simulink model "uGrid_1PH_hd_caso2"  (R2017a)
settings: Solver=VariableStepAuto  StartTime=0.0  StopTime=5  FixedStep=1e-6  MaxStep=1e-4  RelTol=1e-3
PreLoadFcn:
  | SimulinkInit
InitFcn:
  | SimulinkInit
StartFcn:
  | SimulinkInit
StopFcn:
  | EndingScript
values from neighbouring files (symbols this model uses):
  J = 0.3    [SimulinkInit.m]
  K1 = 1.15    [SimulinkInit.m]
  K2 = 1    [SimulinkInit.m]
  K3 = 1    [SimulinkInit.m]
  P = 0.1    [SimulinkInit.m]
  Tao1 = 0.5    [SimulinkInit.m]
  Tao2 = 0.125    [SimulinkInit.m]
undefined symbols (not defined in the file or in its folder): G, GF, Ion, Lithium
libraries: powerlib x56, truetime x15, dsparch4 x12, powerlib_meascontrol x4, electricdrivelib x1, simulink x1
(part 2 of 2)

== system uGrid_1PH_hd_caso2/1Ph_Inverter_bio/Steper3 ==
  In1 : Inport
  Product : Product
  Step : Step  Time=st_time  SampleTime=samp_f
  Out1 : Outport
  wires:
  Product/1 -> Out1/1
  In1/1 -> Product/1
  Step/1 -> Product/2

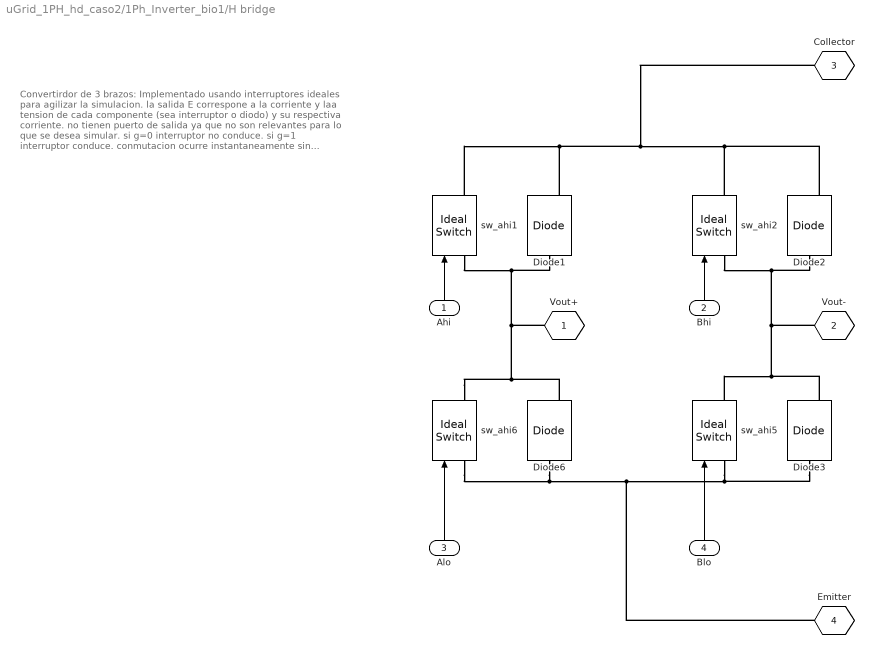
== system uGrid_1PH_hd_caso2/1Ph_Inverter_bio1/H bridge ==
  note: Convertirdor de 3 brazos:
      |
      | Implementado usando interruptores
      | ideales para agilizar la simulacion.
      | la salida E correspone a la corriente y laa
      | tension de cada componente
      | (sea interruptor o diodo) y su respectiva
      | corriente. no tienen puerto de salida ya que no
      | son relevantes para lo que se desea simular.
      |
      | si g=0 interruptor no conduce.
      | si g=1 interruptor conduce.
      |
      | conmutacion ocurre instantaneamente sin
      | retardo.
  Ahi : Inport
  Bhi : Inport  Port=2
  Alo : Inport  Port=3
  Blo : Inport  Port=4
   sw_ahi{1..2,5..6} (4 alike) : powerlib/Power Electronics/Ideal Switch  Ron=0.1  Lon=0  IC=0  Rs=1e6  Cs=10e-12  Measurements=on
  Diode{1..3,6} (4 alike) : powerlib/Power Electronics/Diode  Ron=.2  Lon=0  Vf=0.8  IC=0  UseSnubber=0  Rs=0  Cs=0  Measurements=on
  " Vout+" : PMIOPort  Tag=PMCPort  Port=1  Side=Right
  Vout- : PMIOPort  Tag=PMCPort  Port=2  Side=Right
  Collector : PMIOPort  Tag=PMCPort  Port=3  Side=Right
  Emitter : PMIOPort  Tag=PMCPort  Port=4  Side=Right
  wires:
  Alo/1 -> " sw_ahi6"/1
  Ahi/1 -> " sw_ahi1"/1
  Blo/1 -> " sw_ahi5"/1
  Bhi/1 -> " sw_ahi2"/1
  connections:
  Diode3/RConn1 -- Vout-/RConn1 -- " sw_ahi2"/LConn1 -- Diode2/LConn1 -- " sw_ahi5"/RConn1
  Diode3/LConn1 -- Emitter/RConn1 -- Diode6/LConn1 -- " sw_ahi6"/LConn1 -- " sw_ahi5"/LConn1
  Diode2/RConn1 -- Collector/RConn1 -- " sw_ahi1"/RConn1 -- Diode1/RConn1 -- " sw_ahi2"/RConn1
  " sw_ahi6"/RConn1 -- Diode6/RConn1 -- " Vout+"/RConn1 -- Diode1/LConn1 -- " sw_ahi1"/LConn1

== system uGrid_1PH_hd_caso2/1Ph_Inverter_bio1/Steper1 ==
  In1 : Inport
  Product : Product
  Step : Step  Time=st_time  SampleTime=samp_f
  Out1 : Outport
  wires:
  Step/1 -> Product/2
  In1/1 -> Product/1
  Product/1 -> Out1/1

== system uGrid_1PH_hd_caso2/1Ph_Inverter_bio1/Steper3 ==
  In1 : Inport
  Product : Product
  Step : Step  Time=st_time  SampleTime=samp_f
  Out1 : Outport
  wires:
  Product/1 -> Out1/1
  In1/1 -> Product/1
  Step/1 -> Product/2

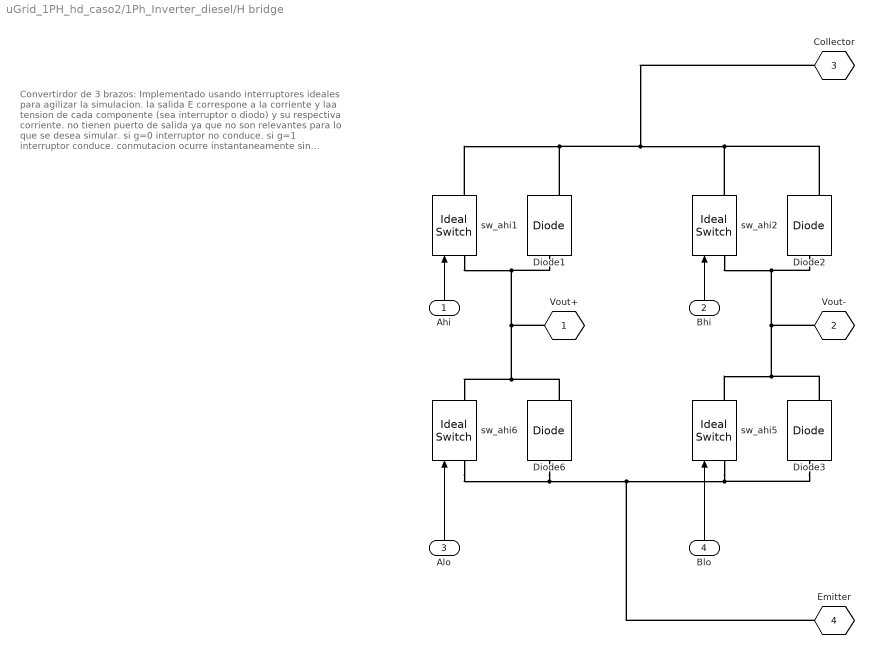
== system uGrid_1PH_hd_caso2/1Ph_Inverter_diesel/H bridge ==
  note: Convertirdor de 3 brazos:
      |
      | Implementado usando interruptores
      | ideales para agilizar la simulacion.
      | la salida E correspone a la corriente y laa
      | tension de cada componente
      | (sea interruptor o diodo) y su respectiva
      | corriente. no tienen puerto de salida ya que no
      | son relevantes para lo que se desea simular.
      |
      | si g=0 interruptor no conduce.
      | si g=1 interruptor conduce.
      |
      | conmutacion ocurre instantaneamente sin
      | retardo.
  Ahi : Inport
  Bhi : Inport  Port=2
  Alo : Inport  Port=3
  Blo : Inport  Port=4
   sw_ahi{1..2,5..6} (4 alike) : powerlib/Power Electronics/Ideal Switch  Ron=0.1  Lon=0  IC=0  Rs=1e6  Cs=10e-12  Measurements=on
  Diode{1..3,6} (4 alike) : powerlib/Power Electronics/Diode  Ron=.2  Lon=0  Vf=0.8  IC=0  UseSnubber=0  Rs=0  Cs=0  Measurements=on
  " Vout+" : PMIOPort  Tag=PMCPort  Port=1  Side=Right
  Vout- : PMIOPort  Tag=PMCPort  Port=2  Side=Right
  Collector : PMIOPort  Tag=PMCPort  Port=3  Side=Right
  Emitter : PMIOPort  Tag=PMCPort  Port=4  Side=Right
  wires:
  Bhi/1 -> " sw_ahi2"/1
  Blo/1 -> " sw_ahi5"/1
  Ahi/1 -> " sw_ahi1"/1
  Alo/1 -> " sw_ahi6"/1
  connections:
  " sw_ahi1"/LConn1 -- Diode1/LConn1 -- " Vout+"/RConn1 -- Diode6/RConn1 -- " sw_ahi6"/RConn1
  " sw_ahi2"/RConn1 -- Diode1/RConn1 -- " sw_ahi1"/RConn1 -- Collector/RConn1 -- Diode2/RConn1
  " sw_ahi5"/LConn1 -- " sw_ahi6"/LConn1 -- Diode6/LConn1 -- Emitter/RConn1 -- Diode3/LConn1
  " sw_ahi5"/RConn1 -- Diode2/LConn1 -- " sw_ahi2"/LConn1 -- Vout-/RConn1 -- Diode3/RConn1

== system uGrid_1PH_hd_caso2/1Ph_Inverter_diesel/Steper1 ==
  In1 : Inport
  Product : Product
  Step : Step  Time=st_time  SampleTime=samp_f
  Out1 : Outport
  wires:
  Product/1 -> Out1/1
  In1/1 -> Product/1
  Step/1 -> Product/2

== system uGrid_1PH_hd_caso2/1Ph_Inverter_diesel/Steper3 ==
  In1 : Inport
  Product : Product
  Step : Step  Time=st_time  SampleTime=samp_f
  Out1 : Outport
  wires:
  Step/1 -> Product/2
  In1/1 -> Product/1
  Product/1 -> Out1/1

== matlab function uGrid_1PH_hd_caso2/1Ph_Inverter_diesel/not_pwm ==
  data: u input; y output
function y = fcn(u)
%#codegen

if(u==0 || u<0)
    a=15;
else
    a=0;
end;

y = a;

== matlab function uGrid_1PH_hd_caso2/1Ph_Inverter_bio/not_pwm ==
  data: u input; y output
function y = fcn(u)
%#codegen

if(u==0 || u<0)
    a=15;
else
    a=0;
end;

y = a;

== matlab function uGrid_1PH_hd_caso2/Optimizador  - Control de tercer nivel/LinProg_BuildMatrices_Reactive_Power ==
  data: H output; Pren_max input; f output; P_load input; K input; A output; lb output; ub output; lbA output; ubA output; Pcsis_max input
function [H, f, A, lb, ub, lbA, ubA] = fcn(Pren_max, P_load, K, Pcsis_max)

% Pr_max es la potencia maxima que puede suministrar el nodo de energias
% renovables.

% P_load es la potencia que consume la carga. ambas potencias son un vector
% de 2 componentes donde la primera componenete es la potencia activa y la
% segunda componenete es la potencia reactiva.

% Kp y Kq corresponde a un vector con los costos de la energia activa y 
% reactiva respectivamente para cada uno de los convertidores, en este caso
% bio y diesel solamente pero pueden agregarse tantas fuentes como se
% desee.

% Pin_max Qin_max corresponde a un vector con los valores maximos de
% potencia activa y reactiva que pueden generar cada una de las otras 
% fuentes diferentes a energias alternativas.


% El bloque qpOASES_(linprog) es un bloque que resuelve el problema standar
% de optimizacion cuadratica :
% 1/2 x' H x + x' f
% sujeto a unas restricciones. la matriz H corresponde a la parte
% cuadratica del problema mientras que f corresponde a la parte lineal. es
% decir que haciendo H = matriz de zeros, es posible reutilizar el bloque
% para solucionar problemas de programacion lineal, que es justamente lo
% que se hace en esta parte del modelo.

% La presente matlab function tiene como tarea formar las matrices f
% y A de restricciones apropiadas para que el bloque de qp oases realice la
% funcione de programacion lineal.

Pm = sum(Pcsis_max); % potencia activa maxima que pueden entregar todas las fuentes (en este caso bio y diesel)


D = P_load - Pren_max; % diferencia entre la potencia que puede generar
% renovables con la que consume la carga.


     % % % % % % % % % % % % % % % % % % % % % % % % % % % % %  
    % Formacion de las entradas para la programacion lineal.  %
     % % % % % % % % % % % % % % % % % % % % % % % % % % % % %  
     
% parte cuadratica de la funcion de coste que se pone en zeros para
% transformarlo en un problema de programacion lineal.
H = zeros(1, length(K)^2);

% funcion de coste lineal.
f = K;

% matriz de restricciones.
% esta formada con la idea de definir que la suma de todas las potencias
% deben almenos cubrir la cantidad de energia activa y reactiva que no
% puede suministrar renovables.
A = ones(1, length(K));

lb = zeros(1, length(K)); % potencia minima que puede generar cada uno de los generadores.
ub = [Pcsis_max]; % potencia maxima que pueden generar cada uno de los generadores.

ubA = [Pm]; % tambien esta relacionado con la potencia min, es un
% requerimiento para el blque de programacion lineal.

% depenediendo la diferencia entre la potencia que pide la carga y la que
% pueden suministrar energias renovables entonces lbA debe establecerce de
% manera conveniente para que el problema de programacion lineal tenga
% solucion.

% restriccion limite inferior para la potencia activa
if(D > 0) % en caso de que renovables no baste para alimentar la carga...
    if(D >= Pm)
        vp = Pm;
    else
        vp = D(1);
    end
else % si renovables basta para alimentar la carga. es decir D = 0 ó negativo
    vp = 0;
end

lbA = vp;

== matlab function uGrid_1PH_hd_caso2/Optimizador  - Control de tercer nivel/LinProg_BuildMatrices_ActivePower ==
  data: H output; Pren_max input; f output; P_load input; K input; A output; lb output; ub output; lbA output; ubA output; Pcsis_max input
function [H, f, A, lb, ub, lbA, ubA] = fcn(Pren_max, P_load, K, Pcsis_max)

% Pr_max es la potencia maxima que puede suministrar el nodo de energias
% renovables.

% P_load es la potencia que consume la carga. ambas potencias son un vector
% de 2 componentes donde la primera componenete es la potencia activa y la
% segunda componenete es la potencia reactiva.

% Kp y Kq corresponde a un vector con los costos de la energia activa y 
% reactiva respectivamente para cada uno de los convertidores, en este caso
% bio y diesel solamente pero pueden agregarse tantas fuentes como se
% desee.

% Pin_max Qin_max corresponde a un vector con los valores maximos de
% potencia activa y reactiva que pueden generar cada una de las otras 
% fuentes diferentes a energias alternativas.


% El bloque qpOASES_(linprog) es un bloque que resuelve el problema standar
% de optimizacion cuadratica :
% 1/2 x' H x + x' f
% sujeto a unas restricciones. la matriz H corresponde a la parte
% cuadratica del problema mientras que f corresponde a la parte lineal. es
% decir que haciendo H = matriz de zeros, es posible reutilizar el bloque
% para solucionar problemas de programacion lineal, que es justamente lo
% que se hace en esta parte del modelo.

% La presente matlab function tiene como tarea formar las matrices f
% y A de restricciones apropiadas para que el bloque de qp oases realice la
% funcione de programacion lineal.

Pm = sum(Pcsis_max); % potencia activa maxima que pueden entregar todas las fuentes (en este caso bio y diesel)


D = P_load - Pren_max; % diferencia entre la potencia que puede generar
% renovables con la que consume la carga.


     % % % % % % % % % % % % % % % % % % % % % % % % % % % % %  
    % Formacion de las entradas para la programacion lineal.  %
     % % % % % % % % % % % % % % % % % % % % % % % % % % % % %  
     
% parte cuadratica de la funcion de coste que se pone en zeros para
% transformarlo en un problema de programacion lineal.
H = zeros(1, length(K)^2);

% funcion de coste lineal.
f = K;

% matriz de restricciones.
% esta formada con la idea de definir que la suma de todas las potencias
% deben almenos cubrir la cantidad de energia activa y reactiva que no
% puede suministrar renovables.
A = ones(1, length(K));

lb = zeros(1, length(K)); % potencia minima que puede generar cada uno de los generadores.
ub = [Pcsis_max]; % potencia maxima que pueden generar cada uno de los generadores.

ubA = [Pm]; % tambien esta relacionado con la potencia min, es un
% requerimiento para el blque de programacion lineal.

% depenediendo la diferencia entre la potencia que pide la carga y la que
% pueden suministrar energias renovables entonces lbA debe establecerce de
% manera conveniente para que el problema de programacion lineal tenga
% solucion.

% restriccion limite inferior para la potencia activa
if(D > 0) % en caso de que renovables no baste para alimentar la carga...
    if(D >= Pm)
        vp = Pm;
    else
        vp = D(1);
    end
else % si renovables basta para alimentar la carga. es decir D = 0 ó negativo
    vp = 0;
end

lbA = vp;

== matlab function uGrid_1PH_hd_caso2/MATLAB Function ==
  data: SOC input; MaxP output; MaxQ output
function [MaxP, MaxQ] = fcn(SOC)


%  funcion que calcula la potencia maxima que puede suministrar las fuentes
%  renovables deacuerdo a la cantidad de carga que hay almancenada en la
%  bateria. esta va de 0 a 100%


% estoc valores que aparecen a continuacion se pusieron de manera
% arbitraria. corresponde a una persona con especialidad en la parte de
% potencia electrica determinar el verdadero algoritmo para hallar la
% potencia que deberia suministrar el nodo de energia renovable deacuerdo a
% la carga de la bateria.

MaxP = 0;
MaxQ = 0;

if( SOC >= 90 )
    MaxP = 500;
    MaxQ = 5000;
end

if( SOC <= 90 )
    MaxP = 200;
    MaxQ = 4000;
end

if( SOC <= 70 )
    MaxP = 100;
    MaxQ = 1000;
end

if( SOC <= 60 )
    MaxP = 50;
    MaxQ = 500;
end

== matlab function uGrid_1PH_hd_caso2/1Ph_Inverter_bio1/not_pwm ==
  data: u input; y output
function y = fcn(u)
%#codegen

if(u==0 || u<0)
    a=15;
else
    a=0;
end;

y = a;

== matlab function uGrid_1PH_hd_caso2/CSI_Control_BIO/MPC_MatCalc ==
  data: ref input; PQ input; Hv output; F output; A output; lb output; ub output; lbA output; ubA output; Du input; MPCout input; G input; GF input
function [Hv, F, A, lb, ub, lbA, ubA] = MPC(ref, PQ, Du, MPCout, G, GF)

%%parametros del MPC


p = 100; % horizonte de prediccion
Nu = 100; % horizonte de control


%% Calculo de la salida de control.

H = G'*G+eye(2*Nu)*3000; % parte cuadratica del qp

ym = [ ones(p, 1)*PQ(1); ones(p, 1)*PQ(2) ]; % vector de la medida de tempearatura actual.

w = [ ones(p, 1)*ref(1); ones(p, 1)*ref(2) ]; % vector señal setpoint.

L = GF*Du+ym; % respuesta libre.

F = 2*(L-w)'*G; % parte lineal del problema qp.

A = zeros(1, 4*Nu*Nu);

lbA = zeros(1, 2*Nu);

ubA = zeros(1, 2*Nu);

Hv = M2V(H);

hip = HiBound(MPCout(1), 600, 10);
hiq = HiBound(MPCout(2), 5000, 1000);

lop = LowBound(MPCout(1), -100, -10);
loq = LowBound(MPCout(2), -100, -1000);

lb = [ones(1, Nu)*lop ones(1, Nu)*loq];
ub = [ones(1, Nu)*hip ones(1, Nu)*hiq];
end

% el control mpc implementado halla mediante programacion cuadratica
% los delta de u optimos deacuerdo a la funcion de coste. por este motivo
% es necesario implementar una logica adicional que permita limitar
% los valores de u (la salida) ya que estos no se manupilan directamente
% en el problema de programacion cuadratica.

% esta logica se implementan en las dos funciones locales que se encuentran
% a continuacion. una funcion define el limite superior y otra funcion para
% definir el limite inferior de los deltas de u deacuerdo al valor actual
% de u para asegurar que tanto los deltas de u como el valor de u esten
% limitados.
% esta funcion solo es correcta si max y Dmax son valores positivos.
function y = HiBound(X, max, Dmax)
    if(X>=0) % si la potencia X es positiva:
        if(max >= X)% si X no ha superado la potencia maxima:
            if(max-X >= Dmax) % si la distancia supera el cambio maximo deseado
                r = Dmax;
            else % si es menor al cambio maximo deseado
                r = max-X;
            end
        else % si X supera la potencia maxima deseada
            r = 0; % el delta maximo es 0 para que no se incremente mas.
        end
    else % si la potencia X es negativa, el incremento maximo es
        r = Dmax;
    end
    y = r;
end

% esta funcion para el lower bound se penso para trbajar con valores
% negativos. si min y Dmin no es negativo la funcion no funciona
% correctamente.
function y = LowBound(X, minv, Dmin)
    if(X<=0) % si la potencia X esta en el cuadrante inferior:
        if(minv <= X)% si X es mayor que la potencia minima:
            if(minv-X <= Dmin) % si la distancia supera el cambio maximo deseado
                r = Dmin;
            else % si es mayor al cambio maximo deseado
                r = minv-X;
            end
        else % si X es menor la potencia maxima deseada
            r = 0; % el delta maximo es 0 para que no se decremente mas.
        end
    else % si la potencia X es positiva, el decremento maximo es
        r = Dmin;
    end
    y = r;
end

== matlab function uGrid_1PH_hd_caso2/CSI_Control_BIO/MPC_OutLogic ==
  data: MPCout output; duv input; Duv output
function [MPCout, Duv] = MPC_out_Logic(duv)

%%parametros del MPC
Nu = 100; % horizonte de control.


%% variables del MPC
persistent Du; % deltas de u 
persistent out; % salida actual del conrolador MPC.

if isempty(Du) % inicializacion de los deltas de uu
    Du = zeros(2*Nu, 1);
end

if isempty(out) % inicializaion de la salida del controlador MPC
    out = [0; 0];
end


du = [duv(1), duv(Nu+1)];


Du = [du(1); Du(1:Nu-1); du(2); Du(Nu+1:end-1)];% actualizar historial deltas de u.

out = [ out(1)+du(1); out(2)+du(2) ]; %calcular salida del controlador.

MPCout = out;
Duv = Du;

== matlab function uGrid_1PH_hd_caso2/CSI_Control_DIESEL/MPC_MatCalc1 ==
  data: ref input; PQ input; Hv output; F output; A output; lb output; ub output; lbA output; ubA output; Du input; MPCout input; G input; GF input
function [Hv, F, A, lb, ub, lbA, ubA] = MPC(ref, PQ, Du, MPCout, G, GF)

%%parametros del MPC


p = 100; % horizonte de prediccion
Nu = 100; % horizonte de control


%% Calculo de la salida de control.

H = G'*G+eye(2*Nu)*3000; % parte cuadratica del qp

ym = [ ones(p, 1)*PQ(1); ones(p, 1)*PQ(2) ]; % vector de la medida de tempearatura actual.

w = [ ones(p, 1)*ref(1); ones(p, 1)*ref(2) ]; % vector señal setpoint.

L = GF*Du+ym; % respuesta libre.

F = 2*(L-w)'*G; % parte lineal del problema qp.

A = zeros(1, 4*Nu*Nu);

lbA = zeros(1, 2*Nu);

ubA = zeros(1, 2*Nu);

Hv = M2V(H);

hip = HiBound(MPCout(1), 600, 10);
hiq = HiBound(MPCout(2), 5000, 1000);

lop = LowBound(MPCout(1), -100, -10);
loq = LowBound(MPCout(2), -100, -1000);

lb = [ones(1, Nu)*lop ones(1, Nu)*loq];
ub = [ones(1, Nu)*hip ones(1, Nu)*hiq];
end

% el control mpc implementado halla mediante programacion cuadratica
% los delta de u optimos deacuerdo a la funcion de coste. por este motivo
% es necesario implementar una logica adicional que permita limitar
% los valores de u (la salida) ya que estos no se manupilan directamente
% en el problema de programacion cuadratica.

% esta logica se implementan en las dos funciones locales que se encuentran
% a continuacion. una funcion define el limite superior y otra funcion para
% definir el limite inferior de los deltas de u deacuerdo al valor actual
% de u para asegurar que tanto los deltas de u como el valor de u esten
% limitados.
% esta funcion solo es correcta si max y Dmax son valores positivos.
function y = HiBound(X, max, Dmax)
    if(X>=0) % si la potencia X es positiva:
        if(max >= X)% si X no ha superado la potencia maxima:
            if(max-X >= Dmax) % si la distancia supera el cambio maximo deseado
                r = Dmax;
            else % si es menor al cambio maximo deseado
                r = max-X;
            end
        else % si X supera la potencia maxima deseada
            r = 0; % el delta maximo es 0 para que no se incremente mas.
        end
    else % si la potencia X es negativa, el incremento maximo es
        r = Dmax;
    end
    y = r;
end

% esta funcion para el lower bound se penso para trbajar con valores
% negativos. si min y Dmin no es negativo la funcion no funciona
% correctamente.
function y = LowBound(X, minv, Dmin)
    if(X<=0) % si la potencia X esta en el cuadrante inferior:
        if(minv <= X)% si X es mayor que la potencia minima:
            if(minv-X <= Dmin) % si la distancia supera el cambio maximo deseado
                r = Dmin;
            else % si es mayor al cambio maximo deseado
                r = minv-X;
            end
        else % si X es menor la potencia maxima deseada
            r = 0; % el delta maximo es 0 para que no se decremente mas.
        end
    else % si la potencia X es positiva, el decremento maximo es
        r = Dmin;
    end
    y = r;
end

== matlab function uGrid_1PH_hd_caso2/CSI_Control_DIESEL/MPC_OutLogic1 ==
  data: MPCout output; duv input; Duv output
function [MPCout, Duv] = MPC_out_Logic(duv)

%%parametros del MPC
Nu = 100; % horizonte de control.


%% variables del MPC
persistent Du; % deltas de u 
persistent out; % salida actual del conrolador MPC.

if isempty(Du) % inicializacion de los deltas de uu
    Du = zeros(2*Nu, 1);
end

if isempty(out) % inicializaion de la salida del controlador MPC
    out = [0; 0];
end


du = [duv(1), duv(Nu+1)];


Du = [du(1); Du(1:Nu-1); du(2); Du(Nu+1:end-1)];% actualizar historial deltas de u.

out = [ out(1)+du(1); out(2)+du(2) ]; %calcular salida del controlador.

MPCout = out;
Duv = Du;
